simulink model "test"  (R2024a)
settings: Solver=VariableStepAuto  StartTime=0.0  StopTime=10.0  RelTol=1e-3
values from neighbouring files (symbols this model uses):
  g = 9.81    [Missile_data.m]
  Missile_mass = 10    [Missile_data.m]
  target_pos = [500, 2000, 1500]    [Missile_data.m]
undefined symbols (not defined in the file or in its folder): deg, rad, s
libraries: simulink x9, aerolibconvert2 x2, shared6dof x1
settings Model: Creator=storm  LastModifiedBy=storm

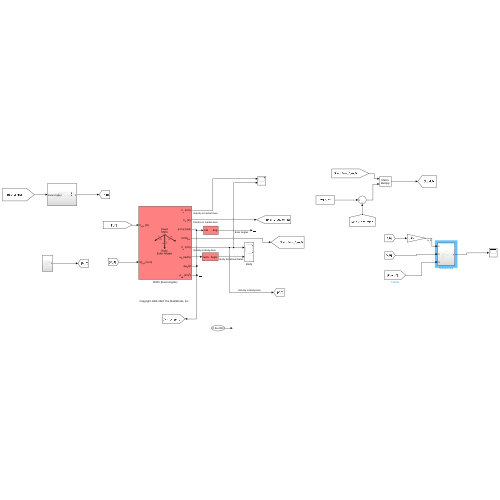
[thumbnail: Simulink's stored preview of the top-level diagram]
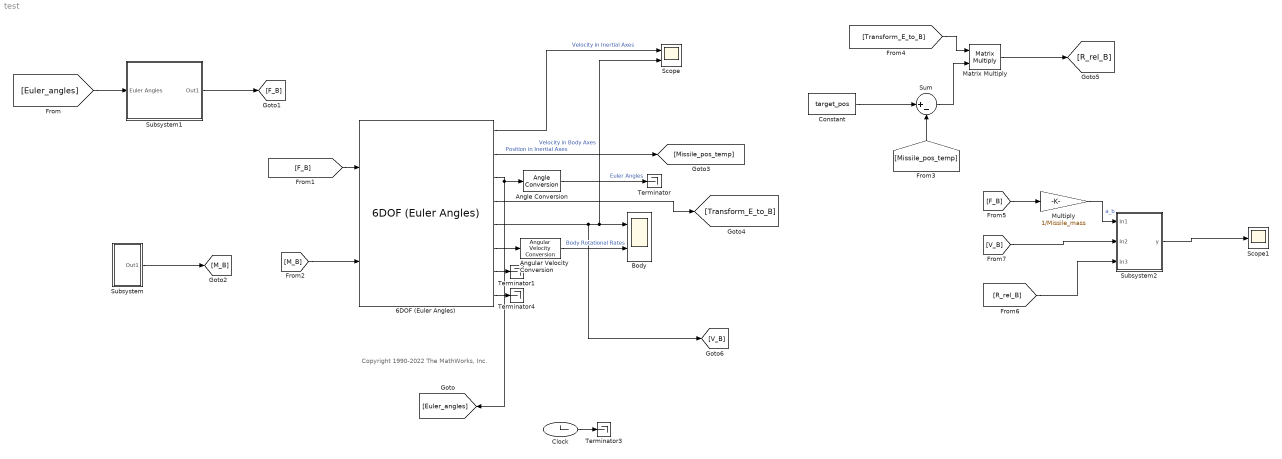
== system test ==
  note: Copyright 1990-2022 The MathWorks, Inc.
  6DOF (Euler Angles) : shared6dof/6DOF (Euler Angles)  units=Metric (MKS)  mtype=Fixed  rep=Euler Angles  xme_0=[0 0 0]  Vm_0=[10 20 30]  eul_0=[0 0 0]  pm_0=[0 0 0]  mass_0=1.0  mass_e=0.5  mass_f=2.0  inertia=eye(3)  inertia_e=eye(3)  inertia_f=2*eye(3)  k_quat=1.0  vre_flag=on  abi_flag=off  aMode=0  xme_statename=''  Vm_statename=''  eul_statename=''  quat_statename=''  pm_statename=''  mass_statename=''
  Angle Conversion : aerolibconvert2/Angle Conversion  IU=rad  OU=deg
  Angular Velocity Conversion : aerolibconvert2/Angular Velocity Conversion  IU=rad/s  OU=deg/s
  Body : Scope  NumInputPorts=2
  Clock : Clock
      settings: Decimation=100
  Constant : Constant  Value=target_pos
  Matrix Multiply : Product  Multiplication=Matrix(*)
  Multiply : Gain  Gain=1/Missile_mass
  Scope : Scope  NumInputPorts=2
  Scope1 : Scope
  Subsystem : Subsystem
  Subsystem1 : Subsystem
  Subsystem2 : Subsystem
  Sum : Sum  Inputs=|+-
  Terminator{,1,3..4} (4 alike) : Terminator
  wires:
  Angular Velocity Conversion/1 -> Body/2  "Body Rotational Rates"
  6DOF (Euler Angles)/3 -> [Euler_angles], Angle Conversion/1
  6DOF (Euler Angles)/1 -> Scope/1  "Velocity in Inertial Axes"
  6DOF (Euler Angles)/7 -> Terminator1/1
  6DOF (Euler Angles)/4 -> [Transform_E_to_B]
  Subsystem1/1(Out1) -> [F_B]
  [Euler_angles] -> Subsystem1/1(Euler Angles)
  6DOF (Euler Angles)/2 -> [Missile_pos_temp]  "Position in Inertial Axes"
  6DOF (Euler Angles)/5 -> [V_B], Scope/2, Body/1  "Velocity in Body Axes"
  6DOF (Euler Angles)/8 -> Terminator4/1
  Clock/1 -> Terminator3/1
  Angle Conversion/1 -> Terminator/1  "Euler Angles"
  6DOF (Euler Angles)/6 -> Angular Velocity Conversion/1
  [F_B] -> 6DOF (Euler Angles)/1
  Subsystem/1(Out1) -> [M_B]
  [M_B] -> 6DOF (Euler Angles)/2
  Constant/1 -> Sum/1
  [Missile_pos_temp] -> Sum/2
  Sum/1 -> Matrix Multiply/2
  [Transform_E_to_B] -> Matrix Multiply/1
  Matrix Multiply/1 -> [R_rel_B]
  [F_B] -> Multiply/1
  [V_B] -> Subsystem2/2(In2)
  [R_rel_B] -> Subsystem2/3(In3)
  Subsystem2/1(y) -> Scope1/1
  Multiply/1 -> Subsystem2/1(In1)  "a_b"

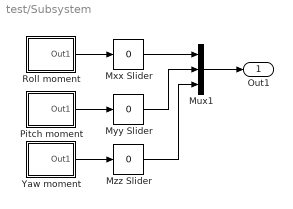
== system test/Subsystem ==
  Mux1 : Mux  Inputs=3
  Mxx Slider : simulink/Math Operations/Slider Gain  gain=0  low=-5  high=10
  Myy Slider : simulink/Math Operations/Slider Gain  gain=0  low=-10  high=10
  Mzz Slider : simulink/Math Operations/Slider Gain  gain=0  low=-1  high=1
  Pitch moment : Subsystem  mask(timed input){t=[0 3 3 4 4 5 5  7.5 7.5 8.5 8.5 9.5 9.5 10], u=[0 0  1 1 -1 -1.005 0 0 -1 -1 1 1 0 0]*3.138/2}
      mask prompts: t "time values:"; u "input values"
      mask Display: plot(t,u)
  Roll moment : Subsystem  mask(timed input){t=[0 1 1 2 2  10], u=[1 1 -1 -.998  0 0]*3.144/2}
      mask prompts: t "time values:"; u "input values"
      mask Display: plot(t,u)
  Yaw moment : Subsystem  mask(timed input){t=[0 6 6 7 7 8 8 10], u=[0 0  -1 -1 1 1 0 0]*3.1/2}
      mask prompts: t "time values:"; u "input values"
      mask Display: plot(t,u)
  Out1 : Outport
  wires:
  Mxx Slider/1 -> Mux1/1
  Pitch moment/1(Out1) -> Myy Slider/1
  Roll moment/1(Out1) -> Mxx Slider/1
  Yaw moment/1(Out1) -> Mzz Slider/1
  Mzz Slider/1 -> Mux1/3
  Myy Slider/1 -> Mux1/2
  Mux1/1 -> Out1/1

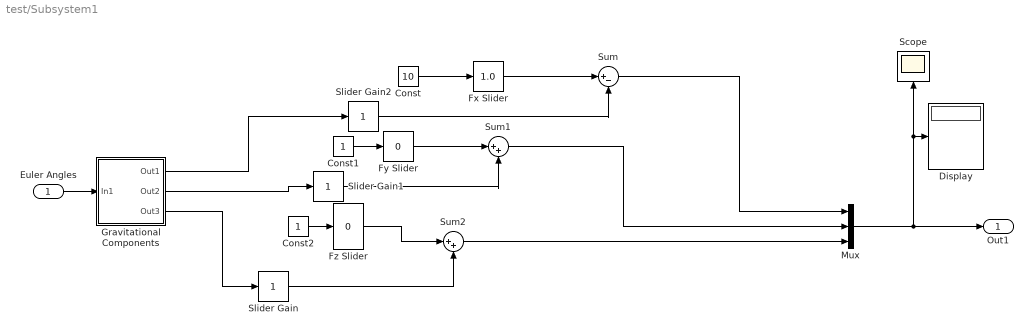
== system test/Subsystem1 ==
  Euler Angles : Inport
  Const : Constant  Value=10
  Const1 : Constant
  Const2 : Constant
  Display : Display
  Fx Slider : simulink/Math Operations/Slider Gain  gain=1.0  low=-1  high=1
  Fy Slider : simulink/Math Operations/Slider Gain  gain=0  low=-1  high=1
  Fz Slider : simulink/Math Operations/Slider Gain  gain=0  low=-1  high=1
  Gravitational Components : Subsystem
  Mux : Mux  Inputs=3
  Scope : Scope
  Slider Gain : simulink/Math Operations/Slider Gain  gain=1  low=0  high=2
  Slider Gain1 : simulink/Math Operations/Slider Gain  gain=1  low=0  high=2
  Slider Gain2 : simulink/Math Operations/Slider Gain  gain=1  low=0  high=2
  Sum : Sum  Inputs=|+-
  Sum1 : Sum  Inputs=|++
  Sum2 : Sum  Inputs=|++
  Out1 : Outport
  wires:
  Fx Slider/1 -> Sum/1
  Const2/1 -> Fz Slider/1
  Mux/1 -> Out1/1, Scope/1, Display/1
  Fy Slider/1 -> Sum1/1
  Const1/1 -> Fy Slider/1
  Const/1 -> Fx Slider/1
  Sum/1 -> Mux/1
  Sum1/1 -> Mux/2
  Fz Slider/1 -> Sum2/1
  Sum2/1 -> Mux/3
  Euler Angles/1 -> Gravitational Components/1(In1)
  Gravitational Components/1(Out1) -> Slider Gain2/1
  Gravitational Components/2(Out2) -> Slider Gain1/1
  Gravitational Components/3(Out3) -> Slider Gain/1
  Slider Gain2/1 -> Sum/2
  Slider Gain1/1 -> Sum1/2
  Slider Gain/1 -> Sum2/2

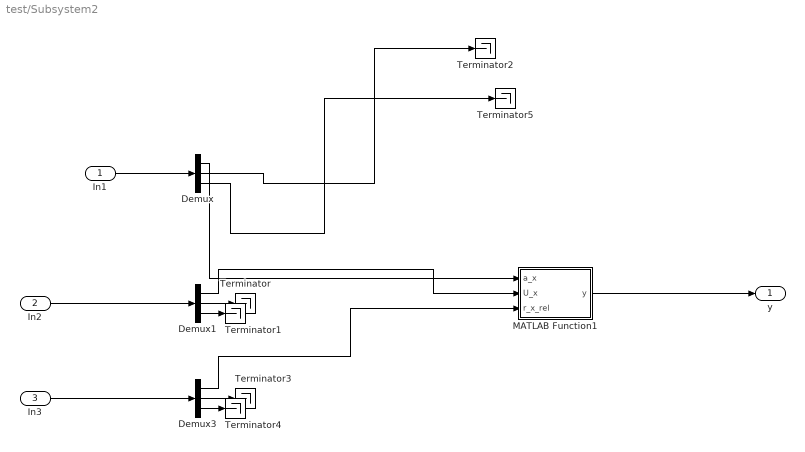
== system test/Subsystem2 ==
  In1 : Inport
  In2 : Inport  Port=2
  In3 : Inport  Port=3
  Demux : Demux  Outputs=3
  Demux1 : Demux  Outputs=3
  Demux3 : Demux  Outputs=3
  MATLAB Function1 : MATLAB Function  TreatAsAtomicUnit=on
  Terminator{,1..5} (6 alike) : Terminator
  y : Outport
  wires:
  Demux1/1 -> MATLAB Function1/2(U_x)
  In2/1 -> Demux1/1
  In1/1 -> Demux/1
  Demux1/2 -> Terminator/1
  Demux/3 -> Terminator5/1
  Demux/2 -> Terminator2/1
  Demux1/3 -> Terminator1/1
  Demux/1 -> MATLAB Function1/1(a_x)
  MATLAB Function1/1(y) -> y/1
  Demux3/3 -> Terminator4/1
  Demux3/1 -> MATLAB Function1/3(r_x_rel)
  In3/1 -> Demux3/1
  Demux3/2 -> Terminator3/1

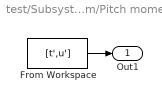
== system test/Subsystem/Pitch moment ==
  From Workspace : FromWorkspace  VariableName=[t',u']  ZeroCross=off
  Out1 : Outport  VectorParamsAs1DForOutWhenUnconnected=off
  wires:
  From Workspace/1 -> Out1/1

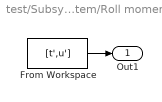
== system test/Subsystem/Roll moment ==
  From Workspace : FromWorkspace  VariableName=[t',u']  ZeroCross=off
  Out1 : Outport  VectorParamsAs1DForOutWhenUnconnected=off
  wires:
  From Workspace/1 -> Out1/1

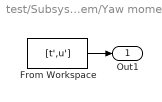
== system test/Subsystem/Yaw moment ==
  From Workspace : FromWorkspace  VariableName=[t',u']  ZeroCross=off
  Out1 : Outport  VectorParamsAs1DForOutWhenUnconnected=off
  wires:
  From Workspace/1 -> Out1/1

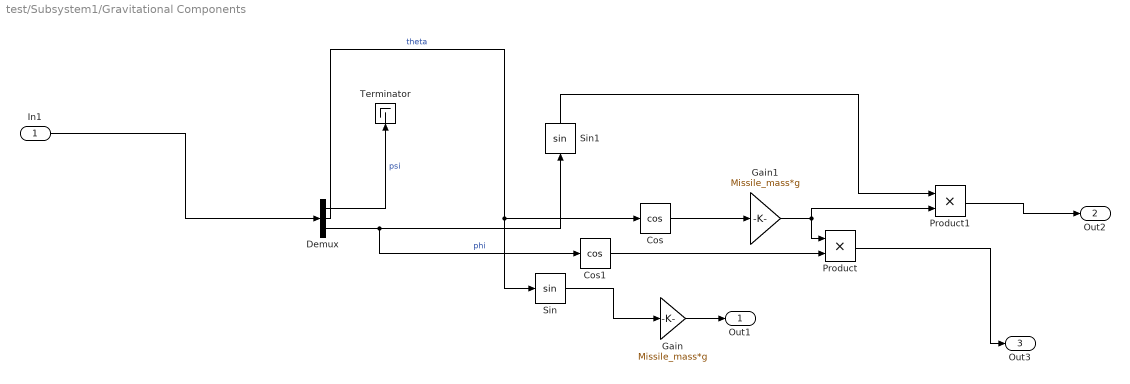
== system test/Subsystem1/Gravitational Components ==
  In1 : Inport
  Cos : Trigonometry  Operator=cos
  Cos1 : Trigonometry  Operator=cos
  Demux : Demux  Outputs=3
  Gain : Gain  Gain=Missile_mass*g
  Gain1 : Gain  Gain=Missile_mass*g
  Product : Product
  Product1 : Product
  Sin : Trigonometry
  Sin1 : Trigonometry
  Terminator : Terminator
  Out1 : Outport
  Out2 : Outport  Port=2
  Out3 : Outport  Port=3
  wires:
  Demux/1 -> Terminator/1  "psi"
  Cos/1 -> Gain1/1
  Cos1/1 -> Product/2
  Product/1 -> Out3/1
  Gain1/1 -> Product/1, Product1/2
  Sin1/1 -> Product1/1
  Demux/2 -> Cos/1, Sin/1  "theta"
  Sin/1 -> Gain/1
  Demux/3 -> Sin1/1, Cos1/1  "phi"
  In1/1 -> Demux/1
  Gain/1 -> Out1/1
  Product1/1 -> Out2/1

== matlab function test/Subsystem2/MATLAB Function1 ==
  data: a_x input; y output; U_x input; r_x_rel input
function y = fcn(a_x, U_x, r_x_rel)
    eq1 = [0.5*a_x, U_x, -r_x_rel];
    r = roots(eq1);
    y = r(2);
    
end
